simulink model "ncp_time_stream_sl"  (R2018b)
settings: Solver=VariableStepAuto  StartTime=0.0  StopTime=10  FixedStep=0.2  RelTol=1e-3  EnableMultiTasking=on
PreLoadFcn:
  | addpath('../')
settings Model: Creator=BK  LastModifiedBy=abartolome
settings DataIOCC: LimitDataPoints=on  SaveFormat=Array
settings OptimizationCC: LifeSpan=inf
settings DebuggingCC: SolverPrmCheckMsg=warning  SFUnexpectedBacktrackingDiag=warning  SFNoUnconditionalDefaultTransitionDiag=warning
settings HardwareCC: ProdBitPerPointer=32  ProdBitPerSizeT=32  ProdBitPerPtrDiffT=32  ProdLargestAtomicFloat=None  ProdIntDivRoundTo=Undefined  ProdEndianess=Unspecified  ProdWordSize=32  ProdHWDeviceType=32-bit Generic
settings ModelReferenceCC: PropagateSignalLabelsOutOfModel=off
settings SFSimCC: SimUseLocalCustomCode=off
settings RTWCC: RTWUseLocalCustomCode=off
settings CodeAppCC: StateflowObjectComments=on
settings GRTTargetCC: TargetLangStandard=C89/C90 (ANSI)  GeneratePreprocessorConditionals=Disable all
settings ConfigComp: CovMetricSettings=dw  CovHtmlReporting=on  CovSaveCumulativeToWorkspaceVar=on  CovSaveSingleToWorkspaceVar=on  CovExternalEMLEnable=off  CovSFcnEnable=off

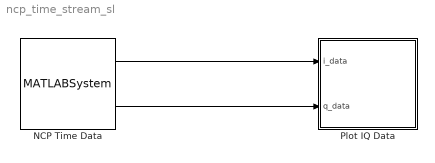
== system ncp_time_stream_sl ==
  NCP Time Data : MATLABSystem  StopFcn=|  System=ncp_time_data  numSamples=10000  centerFreqMHz=900  bandwidthHz=500000  exactMode=1  streaming=0  node_ip=192.0.2.0  node_port=9999  SimulateUsing=Interpreted execution
      | if libisloaded('matlab_ncp_lib')
      |   calllib('matlab_ncp_lib', 'EndTimeCapture');
      |   unloadlibrary('matlab_ncp_lib');
      | end
      mask Type: ncp_time_data
      mask Display:
      | disp('ncp_time_data');
      | port_label('output',1,'i_data');
      | port_label('output',2,'q_data');
  Plot IQ Data : MATLAB Function  TreatAsAtomicUnit=on
  wires:
  NCP Time Data/1 -> Plot IQ Data/1(i_data)
  NCP Time Data/2 -> Plot IQ Data/2(q_data)

== matlab function ncp_time_stream_sl/Plot IQ Data ==
  data: i_data input; q_data input
function plot_iq(i_data,q_data)

% Plot I/Q data
plot(1:length(i_data),i_data(1:length(i_data)),1:length(q_data),q_data(1:length(q_data)));
title('I/Q Data');
xlim([0 length(i_data)]);
ylabel('Voltage \muV');
xlabel('Sample');
